simulink model "pmsm_sysid"  (R2021a)
settings: Solver=VariableStepAuto  StartTime=0.0  StopTime=30  RelTol=1e-3
model workspace (MATLAB code in the model file):
  | np=4; % pole pairs
  | phiv=0.1167; % rotor flux, wb
  | Kt=3/2*np*phiv;
  | f=7.43e-5; %Nm/(rad/s), friction
  | J=1.74e-4; %kgm*m, inertia
  | L=0.004; %H, inductance
  | Ld=L;
  | Lq=L;
  | Rs=1.74; %Ohm, armature resistance
  | Kp=50; % Prop gain in inner PI
  | Ki=2500; % I gain in inner PI
  | Ti = Kp/Ki;
  | h = 1e-2; % Sampling period
  | wN = pi/h; % Nyquist freq
  | wBf = 0.7*wN; % Cutoff freq for AA filter
  | w0f = wBf/2.11; % AA filter param
undefined symbols (not defined in the file or in its folder): den, num
libraries: simulink x2
settings Model: Creator=kjartan  LastModifiedBy=kjartan
settings SolverCC: AlgebraicLoopSolver=TrustRegion
settings DataIOCC: ReturnWorkspaceOutputs=off
settings DebuggingCC: SFMachineParentedDataDiag=warning  ArithmeticOperatorsInVariantConditions=warning
settings SFSimCC: CustomCodeUndefinedFunction=UseInterfaceOnly

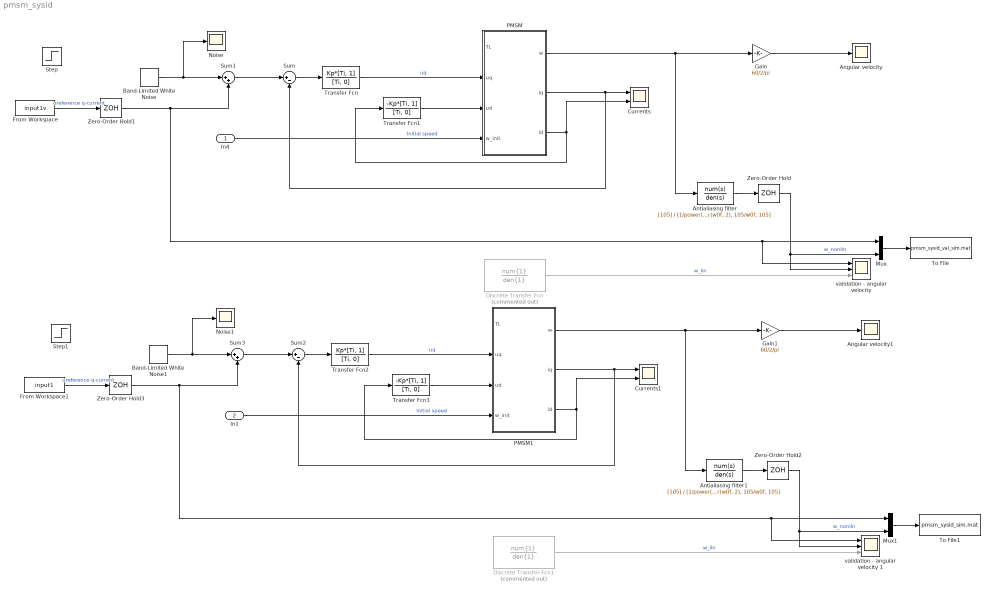
== system pmsm_sysid ==
  In4 : Inport
  In1 : Inport  Port=2
  Angular velocity : Scope
  Angular velocity1 : Scope
  Antialiasing filter : TransferFcn  Numerator=[105]  Denominator=[1/power(w0f,4), 10/power(w0f, 3), 45/power(w0f, 2), 105/w0f, 105]
  Antialiasing filter1 : TransferFcn  Numerator=[105]  Denominator=[1/power(w0f,4), 10/power(w0f, 3), 45/power(w0f, 2), 105/w0f, 105]
  Band-Limited White Noise : simulink/Sources/Band-Limited White Noise  Cov=2  Ts=h  seed=[233412]
  Band-Limited White Noise1 : simulink/Sources/Band-Limited White Noise  Cov=2  Ts=h  seed=[233]
  Currents : Scope  NumInputPorts=2
  Currents1 : Scope  NumInputPorts=2
  Discrete Transfer Fcn : DiscreteTransferFcn  Commented=on  Numerator=num{1}  Denominator=den{1}  SampleTime=h
  Discrete Transfer Fcn1 : DiscreteTransferFcn  Commented=on  Numerator=num{1}  Denominator=den{1}  SampleTime=h
  From Workspace : FromWorkspace  VariableName=input1v  SampleTime=h
  From Workspace1 : FromWorkspace  VariableName=input1  SampleTime=h
  Gain : Gain  Gain=60/2/pi
  Gain1 : Gain  Gain=60/2/pi
  Mux : Mux  Inputs=2
  Mux1 : Mux  Inputs=2
  Noise : Scope
  Noise1 : Scope
  PMSM : Subsystem
  PMSM1 : Subsystem
  Step : Step  After=6  SampleTime=0
  Step1 : Step  After=6  SampleTime=0
  Sum : Sum  Inputs=|+-
  Sum1 : Sum  Inputs=|++
  Sum2 : Sum  Inputs=|+-
  Sum3 : Sum  Inputs=|++
  To File : ToFile  Filename=pmsm_sysid_val_sim.mat  MatrixName=uy  SaveFormat=Timeseries  SampleTime=h
  To File1 : ToFile  Filename=pmsm_sysid_sim.mat  MatrixName=uy  SaveFormat=Timeseries  SampleTime=h
  Transfer Fcn : TransferFcn  Numerator=Kp*[Ti, 1]  Denominator=[Ti, 0]
  Transfer Fcn1 : TransferFcn  Numerator=-Kp*[Ti, 1]  Denominator=[Ti, 0]
  Transfer Fcn2 : TransferFcn  Numerator=Kp*[Ti, 1]  Denominator=[Ti, 0]
  Transfer Fcn3 : TransferFcn  Numerator=-Kp*[Ti, 1]  Denominator=[Ti, 0]
  Zero-Order Hold{,1..3} (4 alike) : ZeroOrderHold  SampleTime=h
  "validation - angular velocity " : Scope  NumInputPorts=3
  validation - angular velocity 1 : Scope  NumInputPorts=3
  wires:
  Transfer Fcn/1 -> PMSM/2(uq)  "uq"
  In4/1 -> PMSM/4(w_init)  "Initial speed"
  PMSM/1(w) -> Gain/1, Antialiasing filter/1
  PMSM/2(iq) -> Sum/2, Currents/1
  PMSM/3(id) -> Currents/2, Transfer Fcn1/1
  Sum/1 -> Transfer Fcn/1
  Transfer Fcn1/1 -> PMSM/3(ud)
  Zero-Order Hold1/1 -> Sum1/2, "validation - angular velocity "/1, Mux/1
  Antialiasing filter/1 -> Zero-Order Hold/1
  Zero-Order Hold/1 -> Mux/2, "validation - angular velocity "/2  "w_nonlin"
  Discrete Transfer Fcn/1 -> "validation - angular velocity "/3  "w_lin"
  Mux/1 -> To File/1
  Gain/1 -> Angular velocity/1
  From Workspace/1 -> Zero-Order Hold1/1  "ureference q-current"
  Band-Limited White Noise/1 -> Noise/1, Sum1/1
  Sum1/1 -> Sum/1
  PMSM1/3(id) -> Currents1/2, Transfer Fcn3/1
  From Workspace1/1 -> Zero-Order Hold3/1  "ureference q-current"
  Band-Limited White Noise1/1 -> Noise1/1, Sum3/1
  In1/1 -> PMSM1/4(w_init)  "Initial speed"
  PMSM1/1(w) -> Gain1/1, Antialiasing filter1/1
  Transfer Fcn2/1 -> PMSM1/2(uq)  "uq"
  Sum3/1 -> Sum2/1
  Sum2/1 -> Transfer Fcn2/1
  Zero-Order Hold3/1 -> Sum3/2, validation - angular velocity 1/1, Mux1/1
  Zero-Order Hold2/1 -> Mux1/2, validation - angular velocity 1/2  "w_nonlin"
  Antialiasing filter1/1 -> Zero-Order Hold2/1
  Discrete Transfer Fcn1/1 -> validation - angular velocity 1/3  "w_lin"
  PMSM1/2(iq) -> Sum2/2, Currents1/1
  Mux1/1 -> To File1/1
  Transfer Fcn3/1 -> PMSM1/3(ud)
  Gain1/1 -> Angular velocity1/1

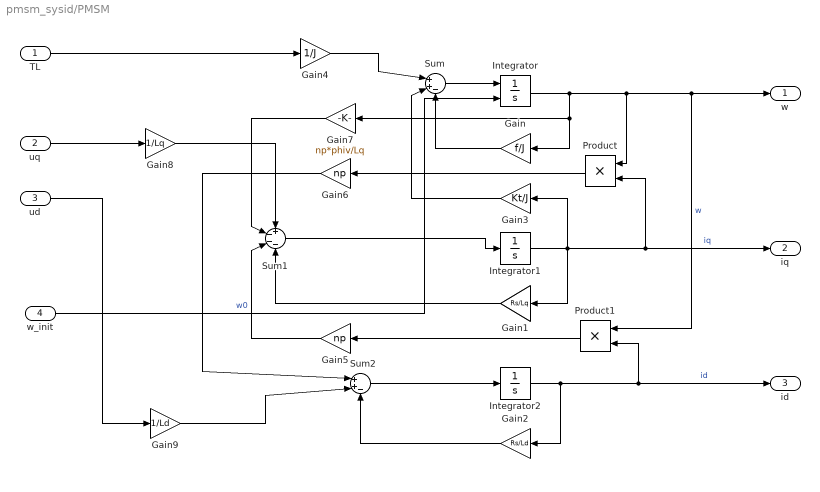
== system pmsm_sysid/PMSM ==
  TL : Inport
  uq : Inport  Port=2
  ud : Inport  Port=3
  w_init : Inport  Port=4
  Gain : Gain  Gain=f/J
  Gain1 : Gain  Gain=Rs/Lq
  Gain2 : Gain  Gain=Rs/Ld
  Gain3 : Gain  Gain=Kt/J
  Gain4 : Gain  Gain=1/J
  Gain5 : Gain  Gain=np
  Gain6 : Gain  Gain=np
  Gain7 : Gain  Gain=np*phiv/Lq
  Gain8 : Gain  Gain=1/Lq
  Gain9 : Gain  Gain=1/Ld
  Integrator : Integrator  InitialConditionSource=external
  Integrator1 : Integrator
  Integrator2 : Integrator
  Product : Product
  Product1 : Product
  Sum : Sum  Inputs=|++-
  Sum1 : Sum  Inputs=+---
  Sum2 : Sum  Inputs=|++-
  w : Outport  VectorParamsAs1DForOutWhenUnconnected=off
  iq : Outport  Port=2  VectorParamsAs1DForOutWhenUnconnected=off
  id : Outport  Port=3  VectorParamsAs1DForOutWhenUnconnected=off
  wires:
  Product/1 -> Gain6/1
  Gain9/1 -> Sum2/2
  Gain2/1 -> Sum2/3
  Gain5/1 -> Sum1/3
  Gain/1 -> Sum/3
  Gain8/1 -> Sum1/1
  Product1/1 -> Gain5/1
  Gain3/1 -> Sum/2
  Gain7/1 -> Sum1/2
  w_init/1 -> Integrator/2  "w0"
  Integrator1/1 -> Gain3/1, Gain1/1, iq/1, Product/2  "iq"
  uq/1 -> Gain8/1
  Sum1/1 -> Integrator1/1
  Integrator/1 -> Gain7/1, Gain/1, Product/1, w/1, Product1/1  "w"
  Gain6/1 -> Sum2/1
  Sum2/1 -> Integrator2/1
  Gain1/1 -> Sum1/4
  Integrator2/1 -> Gain2/1, id/1, Product1/2  "id"
  ud/1 -> Gain9/1
  Sum/1 -> Integrator/1
  TL/1 -> Gain4/1
  Gain4/1 -> Sum/1

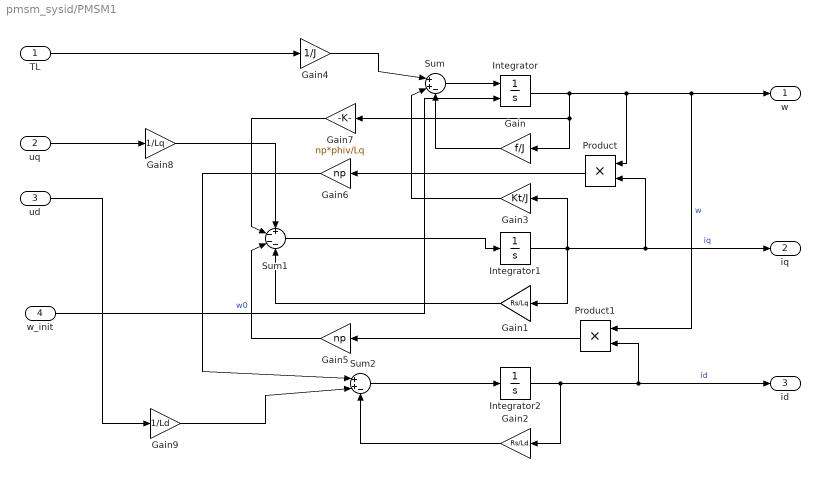
== system pmsm_sysid/PMSM1 ==
  TL : Inport
  uq : Inport  Port=2
  ud : Inport  Port=3
  w_init : Inport  Port=4
  Gain : Gain  Gain=f/J
  Gain1 : Gain  Gain=Rs/Lq
  Gain2 : Gain  Gain=Rs/Ld
  Gain3 : Gain  Gain=Kt/J
  Gain4 : Gain  Gain=1/J
  Gain5 : Gain  Gain=np
  Gain6 : Gain  Gain=np
  Gain7 : Gain  Gain=np*phiv/Lq
  Gain8 : Gain  Gain=1/Lq
  Gain9 : Gain  Gain=1/Ld
  Integrator : Integrator  InitialConditionSource=external
  Integrator1 : Integrator
  Integrator2 : Integrator
  Product : Product
  Product1 : Product
  Sum : Sum  Inputs=|++-
  Sum1 : Sum  Inputs=+---
  Sum2 : Sum  Inputs=|++-
  w : Outport  VectorParamsAs1DForOutWhenUnconnected=off
  iq : Outport  Port=2  VectorParamsAs1DForOutWhenUnconnected=off
  id : Outport  Port=3  VectorParamsAs1DForOutWhenUnconnected=off
  wires:
  Product/1 -> Gain6/1
  Gain9/1 -> Sum2/2
  Gain2/1 -> Sum2/3
  Gain5/1 -> Sum1/3
  Gain/1 -> Sum/3
  Gain8/1 -> Sum1/1
  Product1/1 -> Gain5/1
  Gain3/1 -> Sum/2
  Gain7/1 -> Sum1/2
  w_init/1 -> Integrator/2  "w0"
  Integrator1/1 -> Gain3/1, Gain1/1, iq/1, Product/2  "iq"
  uq/1 -> Gain8/1
  Sum1/1 -> Integrator1/1
  Integrator/1 -> Gain7/1, Gain/1, Product/1, w/1, Product1/1  "w"
  Gain6/1 -> Sum2/1
  Sum2/1 -> Integrator2/1
  Gain1/1 -> Sum1/4
  Integrator2/1 -> Gain2/1, id/1, Product1/2  "id"
  ud/1 -> Gain9/1
  Sum/1 -> Integrator/1
  TL/1 -> Gain4/1
  Gain4/1 -> Sum/1
